simulink model "Noise_Effecr_on_Digital_Transmission"  (R2018a)
settings: Solver=VariableStepAuto  StartTime=0.0  StopTime=5  RelTol=1e-3
libraries: commrandsrc3 x1, dsparch4 x1, commsink2 x1, dspsrcs4 x1, dspsigops x1
settings Model: Creator=ashwin  LastModifiedBy=ashwin

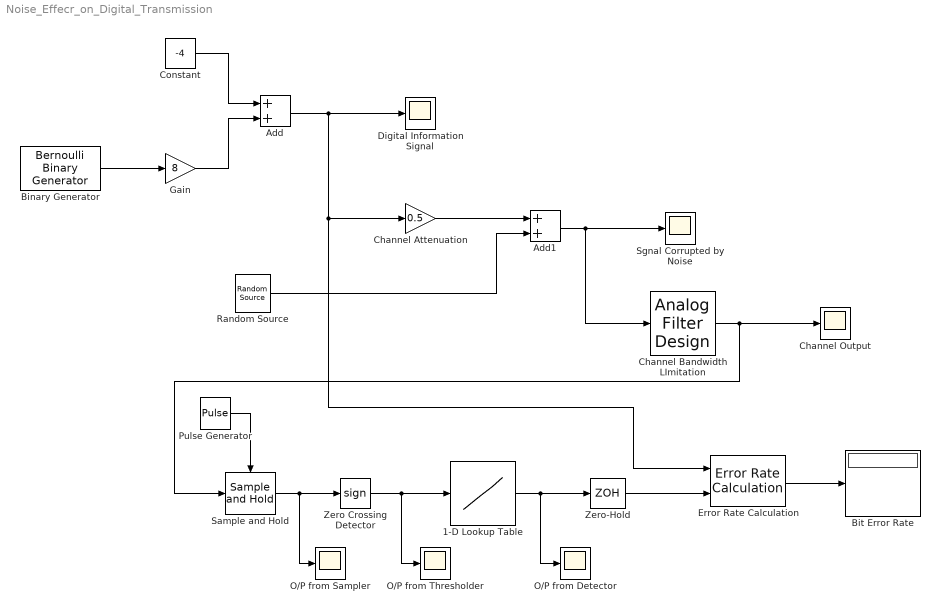
== system Noise_Effecr_on_Digital_Transmission ==
  "1-D Lookup Table " : Lookup_n-D  NumberOfTableDimensions=1  BreakpointsForDimension1=[-1, 1]  Table=[-4, 4]  InternalRulePriority=Speed  RndMeth=Simplest  InputSameDT=on
  Add : Sum
  Add1 : Sum
  Binary Generator : commrandsrc3/Bernoulli Binary Generator  ProbabilityOfZero=0.5  SeedSource=Parameter  Seed=61  SampleTime=0.1  SamplesPerFrame=1  OutputDataType=double  SimulateUsing=Interpreted execution
  Bit Error Rate : Display
  Channel Attenuation : Gain  Gain=0.5
  Channel Bandwidth LImitation : dsparch4/Analog Filter Design  method=Butterworth  filttype=Lowpass  N=10  Wlo=1000  Whi=80  Rp=2  Rs=40
  Channel Output : Scope
  "Constant " : Constant  Value=-4
  Digital Information Signal : Scope
  Error Rate Calculation : commsink2/Error Rate Calculation  N=1  st_delay=0  cp_mode=Entire frame  subframe=[]  PMode=Port  WsName=ErrorVec  RsMode2=off  stop=off  numErr=100  maxBits=1e6
  "Gain " : Gain  Gain=8
  O/P from Detector : Scope
  O/P from Sampler : Scope
  O/P from Thresholder : Scope
  Pulse Generator : DiscretePulseGenerator  PulseType=Time based  Period=0.1  PulseWidth=50
  Random Source : dspsrcs4/Random Source  SrcType=Gaussian  NormMethod=Ziggurat  CltLength=12  MinVal=0  MaxVal=1  MeanVal=0  VarVal=1  RepMode=Not repeatable  rawSeed=1  IsInherit=off  SampMode=Discrete  SampTime=0.01  SampFrame=1  DataType=Double  OutComplex=Real  OutputFrames=off
  Sample and Hold : dspsigops/Sample and Hold  trig=Rising edge  initCond=0  latchinput=off
  Sgnal Corrupted by Noise : Scope
  Zero Crossing Detector : Signum
  Zero-Hold : ZeroOrderHold  SampleTime=0.1
  wires:
  Binary Generator/1 -> "Gain "/1
  "Gain "/1 -> Add/2
  "Constant "/1 -> Add/1
  Add/1 -> Error Rate Calculation/1, Channel Attenuation/1, Digital Information Signal/1
  Channel Attenuation/1 -> Add1/1
  Random Source/1 -> Add1/2
  Add1/1 -> Channel Bandwidth LImitation/1, Sgnal Corrupted by Noise/1
  Channel Bandwidth LImitation/1 -> Sample and Hold/1, Channel Output/1
  Pulse Generator/1 -> Sample and Hold/Trigger
  Sample and Hold/1 -> O/P from Sampler/1, Zero Crossing Detector/1
  Zero Crossing Detector/1 -> O/P from Thresholder/1, "1-D Lookup Table "/1
  "1-D Lookup Table "/1 -> O/P from Detector/1, Zero-Hold/1
  Zero-Hold/1 -> Error Rate Calculation/2
  Error Rate Calculation/1 -> Bit Error Rate/1
